simulink model "windgust_sim"  (R2014b)
settings: Solver=ode45  StartTime=0.0  StopTime=10  RelTol=1e-3
values from neighbouring files (symbols this model uses):
  F = getframe(fig)    [sim_2actuator.m]    (also in simulation.m; simulation_gimbal1.m; simulation_solo.m)
  q = 1/2*1.22*(4.5*340)^2    (= 1427949)    [gimbal_1actuator.m]    (also in gimbal_2actuator.m; part_2.m)
undefined symbols (not defined in the file or in its folder): Light, MIL
libraries: aerolibwind2 x1
settings Model: Creator=Anatole  LastModifiedBy=Anatole

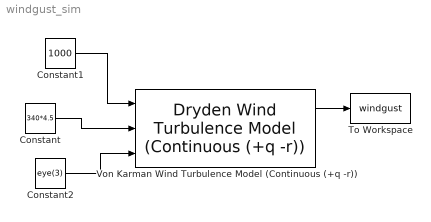
== system windgust_sim ==
  Constant : Constant  Value=340*4.5
  Constant1 : Constant  Value=1000
  Constant2 : Constant  Value=eye(3)
  To Workspace : ToWorkspace  VariableName=windgust  SampleTime=-1
  Von Karman Wind Turbulence Model (Continuous (+q -r)) : aerolibwind2/Dryden Wind Turbulence Model  (Continuous (+q -r))  units=Metric (MKS)  spec=MIL-F-8785C  model=Continuous Von Karman (+q -r)  W20=15  Wdeg=0  TurbProb=10^-2 - Light  L_high=762  Wingspan=10  ts=0.1  Seed=[23341 23342 23343 23344]  T_on=on
  wires:
  Constant/1 -> Von Karman Wind Turbulence Model (Continuous (+q -r))/2
  Constant1/1 -> Von Karman Wind Turbulence Model (Continuous (+q -r))/1
  Constant2/1 -> Von Karman Wind Turbulence Model (Continuous (+q -r))/3
  Von Karman Wind Turbulence Model (Continuous (+q -r))/1 -> To Workspace/1
